simulink model "single_phase_park_transform"  (R2024a)
settings: Solver=VariableStepAuto  StartTime=0.0  StopTime=10.0  RelTol=1e-3
libraries: mcbcontrolslib x1
settings Model: Creator=Administrator  LastModifiedBy=Administrator

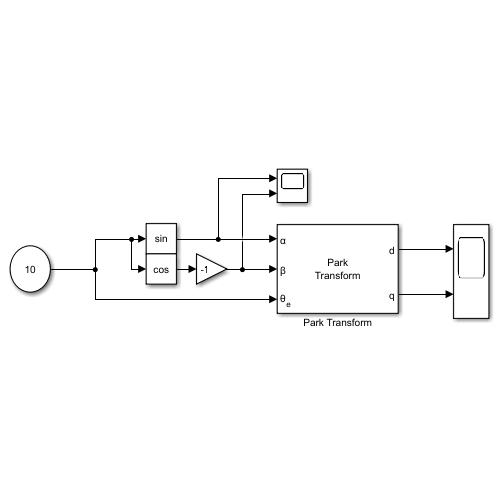
[thumbnail: Simulink's stored preview of the top-level diagram]
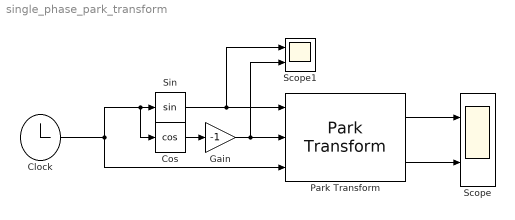
== system single_phase_park_transform ==
  Clock : Clock
  Cos : Trigonometry  Operator=cos
  Gain : Gain  Gain=-1
  Park Transform : mcbcontrolslib/Park Transform  PhaseInput=Two inputs  AxisAlignment=D-axis  ThetaInput=Electrical position  AngleInput=Radians  N_points=1024
      settings: LibrarySourceBlock=mcblib/Controls/Math Transforms/Park Transform
  Scope : Scope  NumInputPorts=2
  Scope1 : Scope  NumInputPorts=2
  Sin : Trigonometry
  wires:
  Park Transform/1 -> Scope/1
  Park Transform/2 -> Scope/2
  Sin/1 -> Scope1/1, Park Transform/1
  Clock/1 -> Park Transform/3, Cos/1, Sin/1
  Cos/1 -> Gain/1
  Gain/1 -> Scope1/2, Park Transform/2
